simulink model "Q_2"  (R2020a)
settings: Solver=FixedStepDiscrete  StartTime=0.0  StopTime=300.0  RelTol=1e-3
undefined symbols (not defined in the file or in its folder): DiscIntNeverNeededParam
libraries: simulink x1, commrandsrc3 x1
settings Model: EnablePacing=on  PacingRate=4  Creator=Admin  LastModifiedBy=Admin

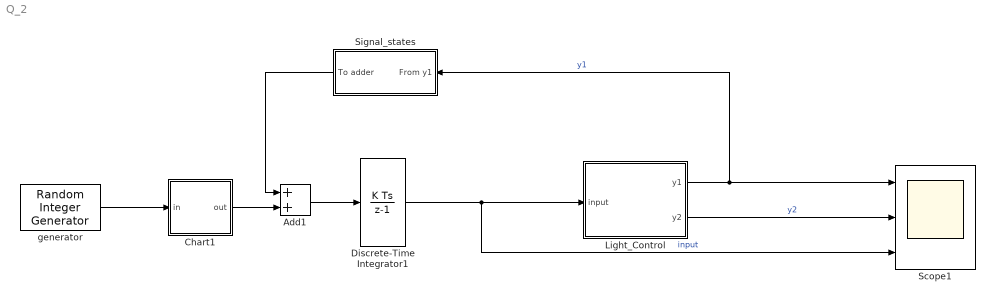
== system Q_2 ==
  Add1 : Sum
  Chart1 : Stateflow chart  TreatAsAtomicUnit=on
  Discrete-Time Integrator1 : DiscreteIntegrator  SampleTime=-1  LimitOutput=on  LowerSaturationLimit=0  ICPrevOutput=DiscIntNeverNeededParam  ICPrevScaledInput=DiscIntNeverNeededParam
  Light_Control : Stateflow chart  TreatAsAtomicUnit=on
  Scope1 : Scope  NumInputPorts=3
  Signal_states : Subsystem  TreatAsAtomicUnit=on
  generator : commrandsrc3/Random Integer Generator  SetSize=100  SeedSource=Auto  Seed=0  SampleTime=0.1  SamplesPerFrame=1  OutputDataType=double  SimulateUsing=Interpreted execution
  wires:
  Light_Control/1(y1) -> Signal_states/1(From y1), Scope1/1  "y1"
  Chart1/1(out) -> Add1/2
  Add1/1 -> Discrete-Time Integrator1/1
  Discrete-Time Integrator1/1 -> Scope1/3, Light_Control/1(input)  "input"
  Signal_states/1(To adder) -> Add1/1
  Light_Control/2(y2) -> Scope1/2  "y2"
  generator/1 -> Chart1/1(in)

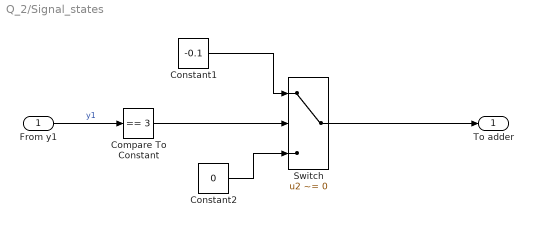
== system Q_2/Signal_states ==
  From y1 : Inport
  Compare To Constant : simulink/Logic and Bit Operations/Compare To Constant  relop===  const=3  OutDataTypeStr=boolean  ZeroCross=off
  Constant1 : Constant  Value=-0.1
  Constant2 : Constant  Value=0
  Switch : Switch  Criteria=u2 ~= 0
  To adder : Outport
  wires:
  Compare To Constant/1 -> Switch/2
  From y1/1 -> Compare To Constant/1  "y1"
  Constant1/1 -> Switch/1
  Switch/1 -> To adder/1
  Constant2/1 -> Switch/3

== stateflow chart Q_2/Chart1 ==
  (default) -> (junction 2) : {out=in>98;}
  data: out output; in input

== stateflow chart Q_2/Light_Control ==
  settings: stateMachineType=MOORE_MACHINE  executeAtInitialization=1  initializeOutput=1
  state Stop
    y1 = RED;
    y2 = GREEN;
  state StopForTraffic
    y1 = RED;
    y2 = GREEN;
  state StopToGo
    y1 = RED;
    y2 = YELLOW;
  state GoToStop
    y1 = YELLOW;
    y2 = RED;
  state Go
    y1 = GREEN;
    y2 = RED;
  (default) -> Stop
  StopForTraffic -> StopToGo : [input]
  Stop -> StopForTraffic : after(20,tick)
  GoToStop -> Stop : after (5,tick)
  StopToGo -> Go : after(5,tick)
  Go -> GoToStop : after(10,tick)
  data: y1 output double; RED constant uint8 =1; YELLOW constant double =2; GREEN constant double =3; y2 output double; input input
